simulink model "CC1"  (Simulink 7.5)
settings: Solver=ode45  StartTime=0.0  StopTime=30  RelTol=1e-3
settings Model: Creator=Fer  LastModifiedBy=Fer

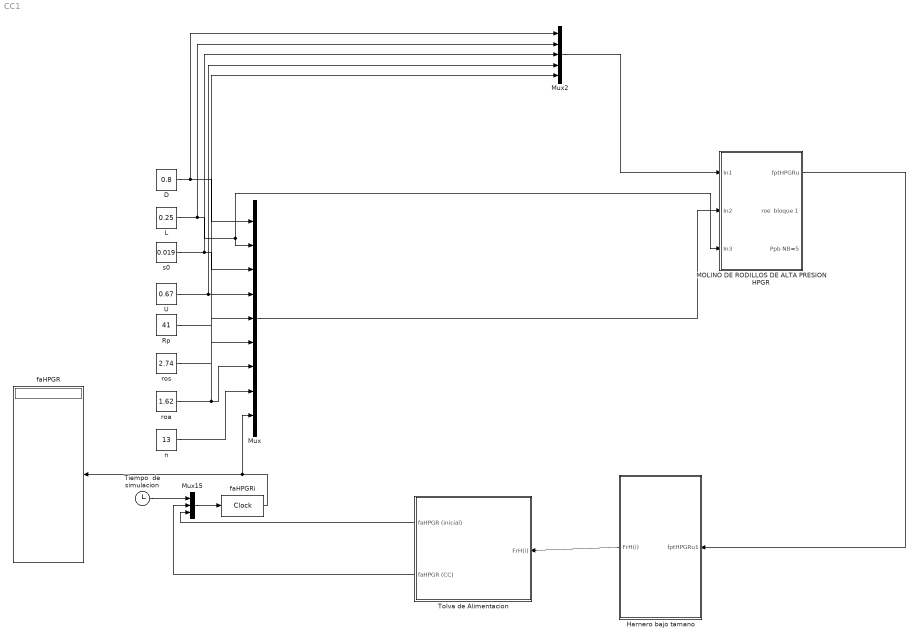
== system CC1 ==
  D : Constant  Value=0.8  OutDataType=fixdt(1, 16)  OutScaling=2^0
  Harnero bajo tamano : Subsystem
  L : Constant  Value=0.25  OutDataType=fixdt(1, 16)  OutScaling=2^0
  MOLINO DE RODILLOS DE ALTA PRESION HPGR : Subsystem
  Mux : Mux  Inputs=9
  Mux15 : Mux  Inputs=3
  Mux2 : Mux  Inputs=5
  Rp : Constant  Value=41  OutDataType=fixdt(1, 16)  OutScaling=2^0
  Tiempo  de simulacion : Clock
      settings: Decimation=10
  Tolva de Alimentacion : Subsystem
  U : Constant  Value=0.67  OutDataType=fixdt(1, 16)  OutScaling=2^0
  faHPGR : Display
  faHPGRi : MATLABFcn  MATLABFcn=Clock
  n : Constant  Value=13  OutDataType=fixdt(1, 16)  OutScaling=2^0
  roa : Constant  Value=1.62  OutDataType=fixdt(1, 16)  OutScaling=2^0
  ros : Constant  Value=2.74  OutDataType=fixdt(1, 16)  OutScaling=2^0
  s0 : Constant  Value=0.019  OutDataType=fixdt(1, 16)  OutScaling=2^0
  wires:
  D/1 -> Mux/1, Mux2/1
  L/1 -> Mux/2, MOLINO DE RODILLOS DE ALTA PRESION HPGR/3(In3), Mux2/2
  s0/1 -> Mux/3, Mux2/3
  U/1 -> Mux/4, Mux2/4
  Rp/1 -> Mux/5
  ros/1 -> Mux/6
  roa/1 -> Mux/7, Mux2/5
  n/1 -> Mux/8
  Mux/1 -> MOLINO DE RODILLOS DE ALTA PRESION HPGR/2(In2)
  Mux2/1 -> MOLINO DE RODILLOS DE ALTA PRESION HPGR/1(In1)
  Tiempo  de simulacion/1 -> Mux15/1
  Mux15/1 -> faHPGRi/1
  Tolva de Alimentacion/2(faHPGR (CC)) -> Mux15/2
  Harnero bajo tamano/1(FrH(i)) -> Tolva de Alimentacion/1(FrH(i))
  Tolva de Alimentacion/1(faHPGR (inicial)) -> Mux15/3
  MOLINO DE RODILLOS DE ALTA PRESION HPGR/1(fptHPGRu) -> Harnero bajo tamano/1(fptHPGRu1)
  faHPGRi/1 -> Mux/9, faHPGR/1

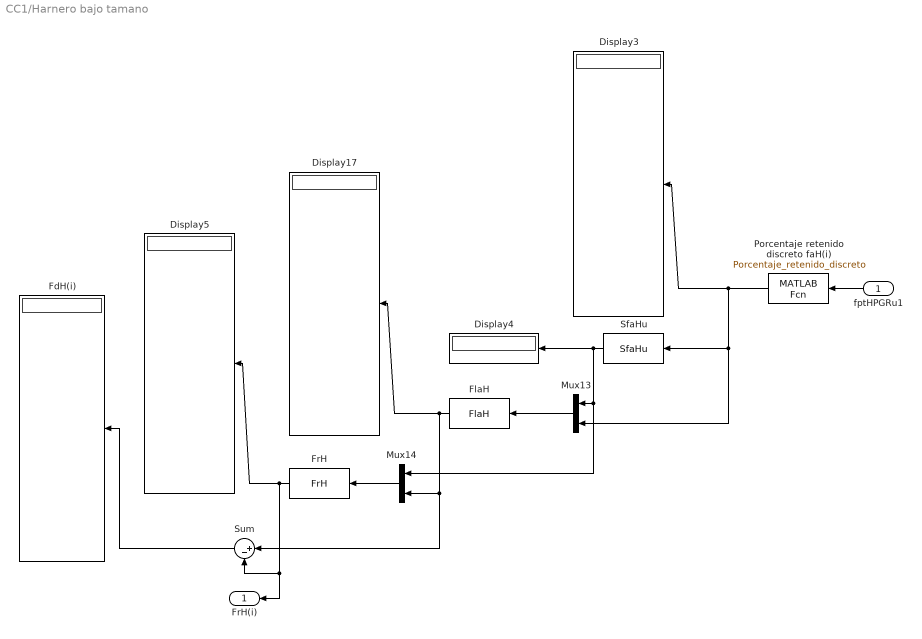
== system CC1/Harnero bajo tamano ==
  fptHPGRu1 : Inport
  Display{3..5,17} (4 alike) : Display
  FdH(i) : Display
  FlaH : MATLABFcn  MATLABFcn=FlaH
  FrH : MATLABFcn  MATLABFcn=FrH
  Mux13 : Mux  Inputs=2
  Mux14 : Mux  Inputs=2
  Porcentaje retenido discreto faH(i) : MATLABFcn  MATLABFcn=Porcentaje_retenido_discreto
  SfaHu : MATLABFcn  MATLABFcn=SfaHu
  Sum : Sum  Inputs=|+-  OutDataType=fixdt(1, 16)  OutScaling=2^0
  FrH(i) : Outport
  wires:
  Porcentaje retenido discreto faH(i)/1 -> Display3/1, SfaHu/1, Mux13/2
  Sum/1 -> FdH(i)/1
  FrH/1 -> Display5/1, FrH(i)/1, Sum/2
  Mux14/1 -> FrH/1
  FlaH/1 -> Display17/1, Mux14/2, Sum/1
  Mux13/1 -> FlaH/1
  SfaHu/1 -> Display4/1, Mux13/1, Mux14/1
  fptHPGRu1/1 -> Porcentaje retenido discreto faH(i)/1

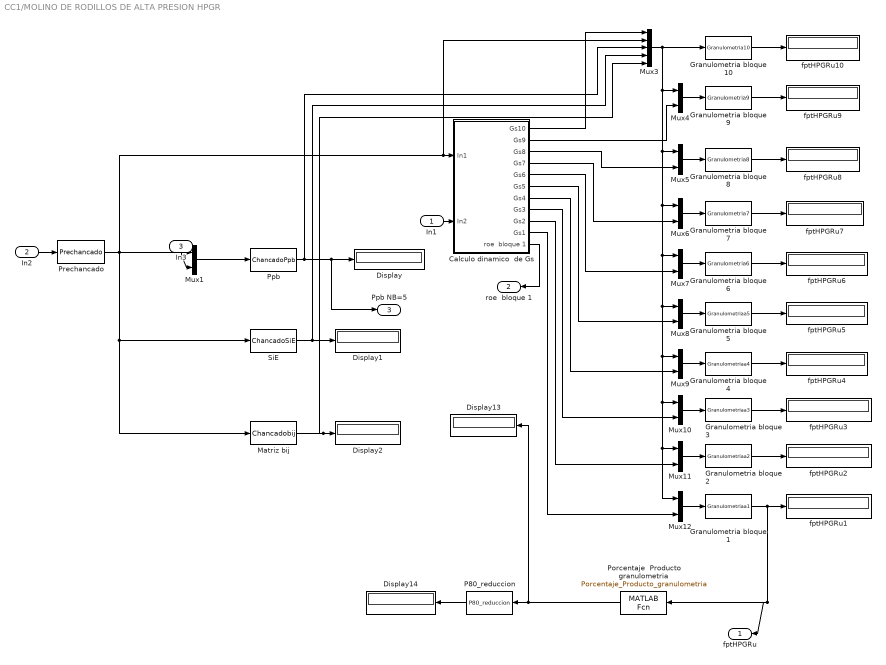
== system CC1/MOLINO DE RODILLOS DE ALTA PRESION HPGR ==
  In1 : Inport
  In2 : Inport  Port=2
  In3 : Inport  Port=3
  Calculo dinamico  de Gs : Subsystem
  Display{,1..2,13..14} (5 alike) : Display
  Granulometria bloque 1 : MATLABFcn  MATLABFcn=Granulometriaa1
  Granulometria bloque 10 : MATLABFcn  MATLABFcn=Granulometria10
  Granulometria bloque 2 : MATLABFcn  MATLABFcn=Granulometriaa2
  Granulometria bloque 3 : MATLABFcn  MATLABFcn=Granulometriaa3
  Granulometria bloque 4 : MATLABFcn  MATLABFcn=Granulometriaa4
  Granulometria bloque 5 : MATLABFcn  MATLABFcn=Granulometriaa5
  Granulometria bloque 6 : MATLABFcn  MATLABFcn=Granulometria6
  Granulometria bloque 7 : MATLABFcn  MATLABFcn=Granulometria7
  Granulometria bloque 8 : MATLABFcn  MATLABFcn=Granulometria8
  Granulometria bloque 9 : MATLABFcn  MATLABFcn=Granulometria9
  Matriz bij : MATLABFcn  MATLABFcn=Chancadobij
  Mux{1,4..12} (10 alike) : Mux  Inputs=2
  Mux3 : Mux  Inputs=5
  P80_reduccion : MATLABFcn  MATLABFcn=P80_reduccion
  Porcentaje  Producto granulometria : MATLABFcn  MATLABFcn=Porcentaje_Producto_granulometria
  Ppb : MATLABFcn  MATLABFcn=ChancadoPpb
  Prechancado : MATLABFcn  MATLABFcn=Prechancado
  SiE : MATLABFcn  MATLABFcn=ChancadoSiE
  fptHPGRu{1..10} (10 alike) : Display
  fptHPGRu : Outport
  roe  bloque 1 : Outport  Port=2
  Ppb NB=5 : Outport  Port=3
  wires:
  Prechancado/1 -> SiE/1, Matriz bij/1, Mux1/1, Calculo dinamico  de Gs/1(In1), Mux3/2
  Mux1/1 -> Ppb/1
  Ppb/1 -> Mux3/3, Display/1, Ppb NB=5/1
  SiE/1 -> Display1/1, Mux3/4
  Matriz bij/1 -> Display2/1, Mux3/5
  Calculo dinamico  de Gs/1(Gs10) -> Mux3/1
  Mux3/1 -> Granulometria bloque 10/1, Mux4/1, Mux5/1, Mux6/1, Mux7/1, Mux8/1, Mux9/1, Mux10/1, Mux11/1, Mux12/1
  Granulometria bloque 10/1 -> fptHPGRu10/1
  Mux4/1 -> Granulometria bloque 9/1
  Calculo dinamico  de Gs/3(Gs8) -> Mux5/2
  Calculo dinamico  de Gs/2(Gs9) -> Mux4/2
  Granulometria bloque 9/1 -> fptHPGRu9/1
  Mux5/1 -> Granulometria bloque 8/1
  Granulometria bloque 8/1 -> fptHPGRu8/1
  Mux6/1 -> Granulometria bloque 7/1
  Granulometria bloque 7/1 -> fptHPGRu7/1
  Calculo dinamico  de Gs/4(Gs7) -> Mux6/2
  Granulometria bloque 6/1 -> fptHPGRu6/1
  Mux7/1 -> Granulometria bloque 6/1
  Calculo dinamico  de Gs/5(Gs6) -> Mux7/2
  Calculo dinamico  de Gs/6(Gs5) -> Mux8/2
  Granulometria bloque 5/1 -> fptHPGRu5/1
  Mux8/1 -> Granulometria bloque 5/1
  Granulometria bloque 4/1 -> fptHPGRu4/1
  Mux9/1 -> Granulometria bloque 4/1
  Calculo dinamico  de Gs/7(Gs4) -> Mux9/2
  Granulometria bloque 3/1 -> fptHPGRu3/1
  Mux10/1 -> Granulometria bloque 3/1
  Calculo dinamico  de Gs/8(Gs3) -> Mux10/2
  Mux11/1 -> Granulometria bloque 2/1
  Calculo dinamico  de Gs/9(Gs2) -> Mux11/2
  Granulometria bloque 1/1 -> Porcentaje  Producto granulometria/1, fptHPGRu/1, fptHPGRu1/1
  Mux12/1 -> Granulometria bloque 1/1
  Calculo dinamico  de Gs/10(Gs1) -> Mux12/2
  Porcentaje  Producto granulometria/1 -> Display13/1, P80_reduccion/1
  P80_reduccion/1 -> Display14/1
  Granulometria bloque 2/1 -> fptHPGRu2/1
  In3/1 -> Mux1/2
  In1/1 -> Calculo dinamico  de Gs/2(In2)
  In2/1 -> Prechancado/1
  Calculo dinamico  de Gs/11(roe  bloque 1) -> roe  bloque 1/1

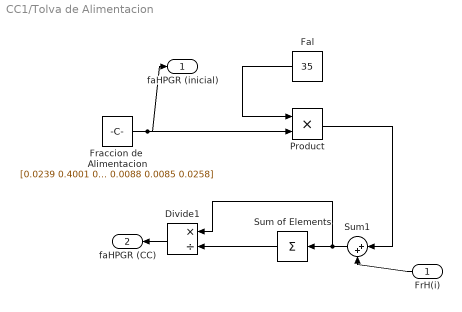
== system CC1/Tolva de Alimentacion ==
  FrH(i) : Inport
  Divide1 : Product  Inputs=*/  OutDataType=fixdt(1, 16)  OutScaling=2^-10
  Fal : Constant  Value=35  OutDataType=fixdt(1, 16)  OutScaling=2^0
  Fraccion de  Alimentacion : Constant  Value=[0.0239 0.4001 0.2089 0.1090 0.0549 0.0441 0.0542 0.0374 0.0159 0.0085 0.0088 0.0085 0.0258]  OutDataType=fixdt(1, 16)  OutScaling=2^0
  Product : Product  OutDataType=fixdt(1, 16)  OutScaling=2^0  RndMeth=Zero
  Sum of Elements : Sum  Inputs=+  OutDataType=fixdt(1, 16)  OutScaling=2^-10
  Sum1 : Sum  Inputs=|++  OutDataType=fixdt(1, 16)  OutScaling=2^0
  faHPGR (inicial) : Outport
  faHPGR (CC) : Outport  Port=2
  wires:
  Fal/1 -> Product/1
  Fraccion de  Alimentacion/1 -> Product/2, faHPGR (inicial)/1
  Product/1 -> Sum1/1
  Sum1/1 -> Sum of Elements/1, Divide1/1
  Sum of Elements/1 -> Divide1/2
  Divide1/1 -> faHPGR (CC)/1
  FrH(i)/1 -> Sum1/2

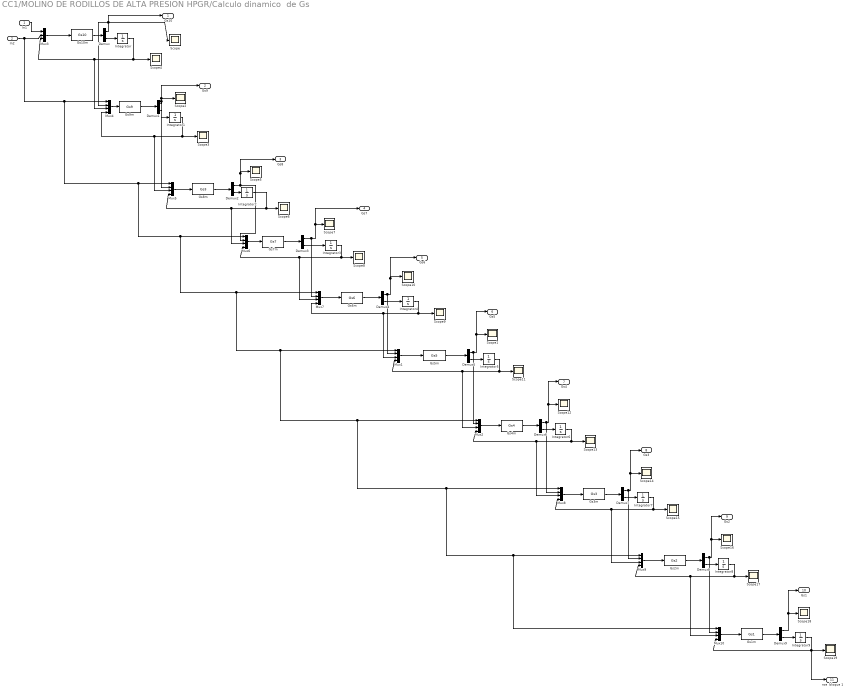
== system CC1/MOLINO DE RODILLOS DE ALTA PRESION HPGR/Calculo dinamico  de Gs ==
  In1 : Inport
  In2 : Inport  Port=2
  Demux{,1..9} (10 alike) : Demux  Outputs=2
  Gs10m : MATLABFcn  MATLABFcn=Gs10
  Gs1m : MATLABFcn  MATLABFcn=Gs1
  Gs2m : MATLABFcn  MATLABFcn=Gs2
  Gs3m : MATLABFcn  MATLABFcn=Gs3
  Gs4m : MATLABFcn  MATLABFcn=Gs4
  Gs5m : MATLABFcn  MATLABFcn=Gs5
  Gs6m : MATLABFcn  MATLABFcn=Gs6
  Gs7m : MATLABFcn  MATLABFcn=Gs7
  Gs8m : MATLABFcn  MATLABFcn=Gs3
  Gs9m : MATLABFcn  MATLABFcn=Gs9
  Integrator{,1..9} (10 alike) : Integrator  InitialCondition=1.6
  Mux{1..2,4..10} (9 alike) : Mux
  Mux3 : Mux  Inputs=3
  Scope{,1..19} (20 alike) : Scope
      Scope1 settings: SaveName=ScopeData10
      Scope10 settings: SaveName=ScopeData9
      Scope11 settings: SaveName=ScopeData11
      Scope12 settings: SaveName=ScopeData12
      Scope13 settings: SaveName=ScopeData13
      Scope14 settings: SaveName=ScopeData14
      Scope15 settings: SaveName=ScopeData15
      Scope16 settings: SaveName=ScopeData16
      Scope17 settings: SaveName=ScopeData17
      Scope18 settings: SaveName=ScopeData18
      Scope19 settings: SaveName=ScopeData19
      Scope3 settings: SaveName=ScopeData2
      Scope4 settings: SaveName=ScopeData3
      Scope5 settings: SaveName=ScopeData4
      Scope6 settings: SaveName=ScopeData5
      Scope7 settings: SaveName=ScopeData6
      Scope8 settings: SaveName=ScopeData7
      Scope9 settings: SaveName=ScopeData8
  Gs10 : Outport  OutDataType=fixdt(1, 16)  OutScaling=2^0
  Gs9 : Outport  Port=2  OutDataType=fixdt(1, 16)  OutScaling=2^0
  Gs8 : Outport  Port=3  OutDataType=fixdt(1, 16)  OutScaling=2^0
  Gs7 : Outport  Port=4  OutDataType=fixdt(1, 16)  OutScaling=2^0
  Gs6 : Outport  Port=5  OutDataType=fixdt(1, 16)  OutScaling=2^0
  Gs5 : Outport  Port=6  OutDataType=fixdt(1, 16)  OutScaling=2^0
  Gs4 : Outport  Port=7  OutDataType=fixdt(1, 16)  OutScaling=2^0
  Gs3 : Outport  Port=8  OutDataType=fixdt(1, 16)  OutScaling=2^0
  Gs2 : Outport  Port=9  OutDataType=fixdt(1, 16)  OutScaling=2^0
  Gs1 : Outport  Port=10  OutDataType=fixdt(1, 16)  OutScaling=2^0
  roe  bloque 1 : Outport  Port=11  OutDataType=fixdt(1, 16)  OutScaling=2^0
  wires:
  In2/1 -> Mux6/1, Mux7/1, Mux1/1, Mux2/1, Mux8/1, Mux9/1, Mux10/1, Mux5/1, Mux4/1, Mux3/2
  Mux3/1 -> Gs10m/1
  Integrator/1 -> Mux3/3, Mux4/3, Scope4/1
  Gs10m/1 -> Demux/1
  Demux/2 -> Integrator/1
  Demux/1 -> Scope/1, Mux4/2, Gs10/1
  Integrator1/1 -> Mux4/4, Mux5/3, Scope3/1
  Demux1/2 -> Integrator1/1
  Mux4/1 -> Gs9m/1
  Gs9m/1 -> Demux1/1
  Demux1/1 -> Mux5/2, Scope2/1, Gs9/1
  Mux5/1 -> Gs8m/1
  Gs8m/1 -> Demux2/1
  Demux2/2 -> Integrator2/1
  Integrator2/1 -> Mux5/4, Mux6/3, Scope6/1
  Demux2/1 -> Mux6/2, Scope5/1, Gs8/1
  Mux6/1 -> Gs7m/1
  Gs7m/1 -> Demux3/1
  Demux3/2 -> Integrator3/1
  Integrator3/1 -> Mux6/4, Mux7/3, Scope8/1
  Demux3/1 -> Mux7/2, Scope7/1, Gs7/1
  Mux7/1 -> Gs6m/1
  Gs6m/1 -> Demux4/1
  Demux4/2 -> Integrator4/1
  Integrator4/1 -> Mux7/4, Mux1/3, Scope9/1
  Demux4/1 -> Scope10/1, Gs6/1, Mux1/2
  In1/1 -> Mux3/1
  Mux1/1 -> Gs5m/1
  Gs5m/1 -> Demux5/1
  Demux5/1 -> Scope1/1, Gs5/1, Mux2/2
  Demux5/2 -> Integrator5/1
  Integrator5/1 -> Mux1/4, Mux2/3, Scope11/1
  Mux2/1 -> Gs4m/1
  Gs4m/1 -> Demux6/1
  Demux6/2 -> Integrator6/1
  Demux6/1 -> Scope12/1, Gs4/1, Mux8/2
  Integrator6/1 -> Mux2/4, Mux8/3, Scope13/1
  Mux8/1 -> Gs3m/1
  Gs3m/1 -> Demux7/1
  Demux7/1 -> Scope14/1, Gs3/1, Mux9/2
  Demux7/2 -> Integrator7/1
  Integrator7/1 -> Mux8/4, Mux9/3, Scope15/1
  Gs2m/1 -> Demux8/1
  Demux8/1 -> Scope16/1, Gs2/1, Mux10/2
  Demux8/2 -> Integrator8/1
  Integrator8/1 -> Mux9/4, Mux10/3, Scope17/1
  Mux9/1 -> Gs2m/1
  Mux10/1 -> Gs1m/1
  Gs1m/1 -> Demux9/1
  Demux9/1 -> Scope18/1, Gs1/1
  Demux9/2 -> Integrator9/1
  Integrator9/1 -> Mux10/4, Scope19/1, roe  bloque 1/1
